simulink model "SW_Avionic"  (R2020a)
settings: Solver=FixedStepAuto  StartTime=0.0  StopTime=inf  FixedStep=0.01  RelTol=1e-3  EnableMultiTasking=on
libraries: bbblueCommlib x31, svdutilitieslib x13, bbblueBasicLib x6, bbblueSensorLib x3, simulink x1
settings Model: ExtModeTrigDuration=100  Creator=sokserey  LastModifiedBy=ASUS
settings SolverCC: PositivePriorityOrder=on  AutoInsertRateTranBlk=on
settings OptimizationCC: EnhancedBackFolding=on  PassReuseOutputArgsAs=Individual arguments  ZeroExternalMemoryAtStartup=off  ZeroInternalMemoryAtStartup=off  MaxStackSize=64  OptimizeBlockOrder=speed  DifferentSizesBufferReuse=on  OptimizationCustomize=off  EfficientTunableParamExpr=on
settings DebuggingCC: ParameterTunabilityLossMsg=error  SFMachineParentedDataDiag=error
settings HardwareCC: ProdBitPerPointer=32  ProdBitPerSizeT=32  ProdBitPerPtrDiffT=32  ProdLargestAtomicInteger=Long  ProdLargestAtomicFloat=Double  ProdWordSize=32  ProdHWDeviceType=ARM Compatible->ARM Cortex
settings SFSimCC: MATLABDynamicMemAlloc=off
settings RTWCC: SystemTargetFile=ert.tlc  HardwareBoard=BeagleBone Blue  TemplateMakefile=ert_default_tmf  Toolchain=GNU GCC BeagleBone Blue
settings CodeAppCC: ForceParamTrailComments=on  IgnoreCustomStorageClasses=off  OperatorAnnotations=on  SimulinkDataObjDesc=on  SFDataObjDesc=on  InsertBlockDesc=on
settings ERTTargetCC: SupportContinuousTime=on  SupportVariableSizeSignals=on

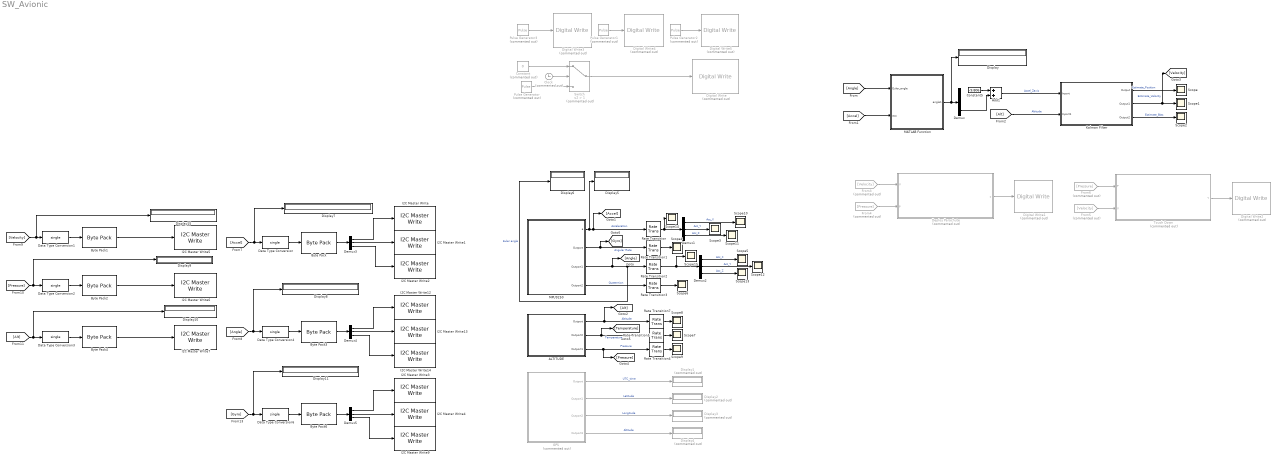
== system SW_Avionic ==
  "ALTITUDE " : Subsystem
  Add1 : Sum
  Byte Pack{,1..4,6} (6 alike) : svdutilitieslib/Byte Pack  maskPackedDataType=uint8  datatypes={'single'}  byteAlign=1  blockPlatform=arduinoert
      settings: SourceProductBaseCode=ARDUINO,ML_ARDUINO,ECCORTEXA,ECCORTEXR,SC_BEAGLEBONE_BLUE,EC_FREEDOM_BOARD,EC_FRDM_K64F,INTEL_BLOCKSET,MICROBIT,NUCLEO,PX4AUTOPILOTS,RASPPIIO,STMICRODIS,TIC2000,XILINX_BLOCKSET
  Clock : Clock  Commented=on
  Constant : Constant  Commented=on  Value=0
  Constant5 : Constant  Value=-9.806
  Data Type Conversion{,1..4,6} (6 alike) : DataTypeConversion  OutDataTypeStr=single
  Demux{,1..5} (6 alike) : Demux  Outputs=3
  "Deploy Parachute " : Stateflow chart  Commented=on  TreatAsAtomicUnit=on
  Digital Write : bbblueBasicLib/Digital Write  Commented=on  GPIOSelect=GPIO3_17  Pin=49  Direction=output
      settings: SourceProductBaseCode=SC_BEAGLEBONE_BLUE
  Digital Write1 : bbblueBasicLib/Digital Write  Commented=on  GPIOSelect=GPIO3_2  Pin=49  Direction=output
      settings: SourceProductBaseCode=SC_BEAGLEBONE_BLUE
  Digital Write2 : bbblueBasicLib/Digital Write  Commented=on  GPIOSelect=GPIO3_1  Pin=49  Direction=output
      settings: SourceProductBaseCode=SC_BEAGLEBONE_BLUE
  Digital Write3 : bbblueBasicLib/Digital Write  Commented=on  GPIOSelect=GPIO1_25  Pin=49  Direction=output
      settings: SourceProductBaseCode=SC_BEAGLEBONE_BLUE
  Digital Write4 : bbblueBasicLib/Digital Write  Commented=on  GPIOSelect=GPIO1_17  Pin=49  Direction=output
      settings: SourceProductBaseCode=SC_BEAGLEBONE_BLUE
  Digital Write5 : bbblueBasicLib/Digital Write  Commented=on  GPIOSelect=GPIO3_20  Pin=49  Direction=output
      settings: SourceProductBaseCode=SC_BEAGLEBONE_BLUE
  Display{,5..11,15} (9 alike) : Display
  Display{1..4} (4 alike) : Display  Commented=on
  From3 : From  Commented=on  GotoTag=Velocity
  From4 : From  Commented=on  GotoTag=Pressure
  From5 : From  Commented=on  GotoTag=Velocity
  From6 : From  Commented=on  GotoTag=Pressure
  GPS : Subsystem  Commented=on
  I2C Master Write{,1..7,9,12..14} (12 alike) : bbblueCommlib/I2C Master Write  I2CModule=1  Mode=Master  SlaveAddress=8  SlaveByteOrder=BigEndian  Direction=Transmitter  RegisterAddressMode=off  RegisterAddress=0  SlaveDataType=uint8  DataLength=1  NoAck=off  RepeatedStart=off  OutputStatus=off
      settings: SourceProductBaseCode=SC_BEAGLEBONE_BLUE
  "Kalman Filter " : Subsystem
  MATLAB Function : MATLAB Function  TreatAsAtomicUnit=on
  MPU9250 : Subsystem
  Pulse Generator : DiscretePulseGenerator  Commented=on  PulseType=Time based  Period=0.5  PulseWidth=50  VectorParams1D=off
  Pulse Generator1 : DiscretePulseGenerator  Commented=on  PulseType=Time based  Period=1  PulseWidth=33  PhaseDelay=0.33
  Pulse Generator2 : DiscretePulseGenerator  Commented=on  PulseType=Time based  Period=1  PulseWidth=33  PhaseDelay=0.66  VectorParams1D=off
  Pulse Generator3 : DiscretePulseGenerator  Commented=on  PulseType=Time based  Period=1  PulseWidth=33  VectorParams1D=off
  Rate Transition{,1..3} (4 alike) : RateTransition  OutPortSampleTime=0.01
  Rate Transition4 : RateTransition  OutPortSampleTime=0.1
  Rate Transition5 : RateTransition  OutPortSampleTime=0.1
  Rate Transition7 : RateTransition  OutPortSampleTime=0.1
  Scope{,1..15} (16 alike) : Scope
  Switch : Switch  Commented=on  Criteria=u2 > Threshold  Threshold=1
  "Touch Down " : Stateflow chart  Commented=on  TreatAsAtomicUnit=on
  wires:
  Clock/1 -> Switch/2
  Constant/1 -> Switch/1
  Pulse Generator/1 -> Switch/3
  Switch/1 -> Digital Write/1
  MPU9250/3(Outport1) -> Display6/1, Rate Transition2/1, [Angle]  "Euler angle"
  MPU9250/2(Outport) -> [Gyro], Rate Transition1/1  "Angular Rate"
  MPU9250/1(a) -> Rate Transition/1, [Accel], Display5/1  "Acceleration"
  MPU9250/4(Outport2) -> Rate Transition3/1  "Quaternion"
  "ALTITUDE "/3(Outport1) -> Rate Transition4/1, [Pressure]  "Pressure"
  Pulse Generator2/1 -> Digital Write5/1
  Pulse Generator1/1 -> Digital Write4/1
  Pulse Generator3/1 -> Digital Write3/1
  Constant5/1 -> Add1/1
  Add1/1 -> "Kalman Filter "/1(Inport)  "Accel_Zaxis"
  "Kalman Filter "/1(Output) -> Scope/1  "Estimate_Position"
  "Kalman Filter "/2(Output1) -> [Velocity], Scope1/1  "Estimate_Velocity"
  "Kalman Filter "/3(Output2) -> Scope2/1  "Estimate_Bias"
  [Angle] -> MATLAB Function/1(Euler_angle)
  [Accel] -> MATLAB Function/2(acc)
  MATLAB Function/1(angle1) -> Display/1, Demux/1
  Demux/3 -> Add1/2
  [Alt] -> "Kalman Filter "/2(Inport1)  "Altitude"
  GPS/1(Outport) -> Display1/1  "UTC_time"
  GPS/2(Outport1) -> Display2/1  "Latitude"
  GPS/3(Outport2) -> Display3/1  "Longitude"
  GPS/4(Outport3) -> Display4/1  "Altitude"
  Rate Transition1/1 -> Scope4/1
  Rate Transition3/1 -> Scope6/1
  Rate Transition7/1 -> Scope8/1
  Rate Transition5/1 -> Scope7/1
  Rate Transition4/1 -> Scope9/1
  "ALTITUDE "/1(Outport) -> [Alt], Rate Transition7/1  "Altitude"
  "ALTITUDE "/2(Outport2) -> [Temperature], Rate Transition5/1  "Temperature"
  "Deploy Parachute "/1(y) -> Digital Write1/1
  From3/1 -> "Deploy Parachute "/1(V)
  From4/1 -> "Deploy Parachute "/2(P)
  From5/1 -> "Touch Down "/2(V)
  From6/1 -> "Touch Down "/1(P)
  "Touch Down "/1(Y) -> Digital Write2/1
  Rate Transition/1 -> Scope14/1, Demux1/1
  Demux1/1 -> Scope10/1  "Acc_X"
  Demux1/2 -> Scope3/1  "Acc_Y"
  Demux1/3 -> Scope11/1  "Acc_Z"
  Rate Transition2/1 -> Scope15/1, Demux2/1
  Demux2/1 -> Scope5/1  "Acc_X"
  Demux2/3 -> Scope13/1  "Acc_Z"
  Demux2/2 -> Scope12/1  "Acc_Y"
  Demux3/3 -> I2C Master Write2/1
  Data Type Conversion4/1 -> Byte Pack3/1
  Byte Pack/1 -> Demux3/1
  Demux3/2 -> I2C Master Write1/1
  Demux4/3 -> I2C Master Write14/1
  Byte Pack3/1 -> Demux4/1
  Demux4/1 -> I2C Master Write12/1
  Demux4/2 -> I2C Master Write13/1
  Data Type Conversion/1 -> Byte Pack/1
  Demux3/1 -> I2C Master Write/1
  [Accel] -> Display7/1, Data Type Conversion/1
  [Angle] -> Display8/1, Data Type Conversion4/1
  Data Type Conversion1/1 -> Byte Pack1/1
  [Velocity] -> Display15/1, Data Type Conversion1/1
  Data Type Conversion2/1 -> Byte Pack2/1
  Byte Pack2/1 -> I2C Master Write6/1
  [Pressure] -> Display9/1, Data Type Conversion2/1
  Byte Pack4/1 -> I2C Master Write7/1
  [Alt] -> Display10/1, Data Type Conversion3/1
  Data Type Conversion3/1 -> Byte Pack4/1
  Byte Pack1/1 -> I2C Master Write5/1
  Demux5/1 -> I2C Master Write3/1
  [Gyro] -> Display11/1, Data Type Conversion6/1
  Byte Pack6/1 -> Demux5/1
  Demux5/2 -> I2C Master Write4/1
  Demux5/3 -> I2C Master Write9/1
  Data Type Conversion6/1 -> Byte Pack6/1

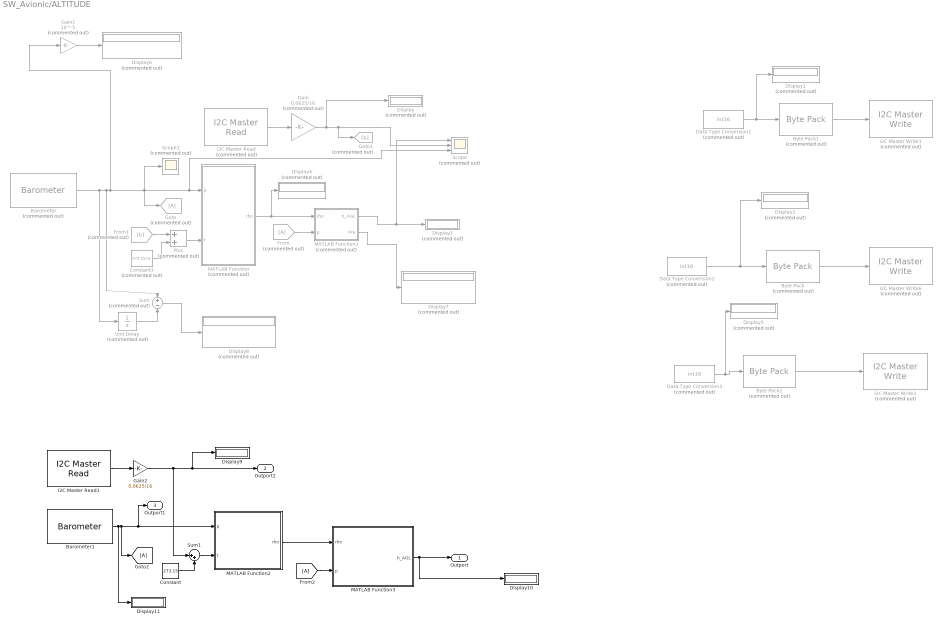
== system SW_Avionic/ALTITUDE  ==
  Barometer : bbblueSensorLib/Barometer  Commented=on  OSRSelection=16  IIRFilterCoeff=16  SampleTime=0.01
      settings: SourceProductBaseCode=SC_BEAGLEBONE_BLUE
  Barometer1 : bbblueSensorLib/Barometer  OSRSelection=16  IIRFilterCoeff=16  SampleTime=0.01
      settings: SourceProductBaseCode=SC_BEAGLEBONE_BLUE
  Byte Pack : svdutilitieslib/Byte Pack  Commented=on  maskPackedDataType=uint8  datatypes={'int16'}  byteAlign=1  blockPlatform=arduinoert
      settings: SourceProductBaseCode=ARDUINO,ML_ARDUINO,ECCORTEXA,ECCORTEXR,SC_BEAGLEBONE_BLUE,EC_FREEDOM_BOARD,EC_FRDM_K64F,INTEL_BLOCKSET,MICROBIT,NUCLEO,PX4AUTOPILOTS,RASPPIIO,STMICRODIS,TIC2000,XILINX_BLOCKSET
  Byte Pack1 : svdutilitieslib/Byte Pack  Commented=on  maskPackedDataType=uint8  datatypes={'int16'}  byteAlign=1  blockPlatform=arduinoert
      settings: SourceProductBaseCode=ARDUINO,ML_ARDUINO,ECCORTEXA,ECCORTEXR,SC_BEAGLEBONE_BLUE,EC_FREEDOM_BOARD,EC_FRDM_K64F,INTEL_BLOCKSET,MICROBIT,NUCLEO,PX4AUTOPILOTS,RASPPIIO,STMICRODIS,TIC2000,XILINX_BLOCKSET
  Byte Pack2 : svdutilitieslib/Byte Pack  Commented=on  maskPackedDataType=uint8  datatypes={'int16'}  byteAlign=1  blockPlatform=arduinoert
      settings: SourceProductBaseCode=ARDUINO,ML_ARDUINO,ECCORTEXA,ECCORTEXR,SC_BEAGLEBONE_BLUE,EC_FREEDOM_BOARD,EC_FRDM_K64F,INTEL_BLOCKSET,MICROBIT,NUCLEO,PX4AUTOPILOTS,RASPPIIO,STMICRODIS,TIC2000,XILINX_BLOCKSET
  Constant : Constant  Value=273.15
  Constant3 : Constant  Commented=on  Value=273.15+6
  Data Type Conversion1 : DataTypeConversion  Commented=on  OutDataTypeStr=int16
  Data Type Conversion2 : DataTypeConversion  Commented=on  OutDataTypeStr=int16
  Data Type Conversion3 : DataTypeConversion  Commented=on  OutDataTypeStr=int16
  Display{,1..8} (9 alike) : Display  Commented=on
  Display10 : Display
  Display11 : Display
  Display9 : Display
  From : From  Commented=on
  From1 : From  Commented=on  GotoTag=b
  Gain : Gain  Commented=on  Gain=0.0625/16  OutDataTypeStr=single
  Gain1 : Gain  Commented=on  Gain=10^-5
  Gain2 : Gain  Gain=0.0625/16  OutDataTypeStr=single
  Goto : Goto  Commented=on
  Goto1 : Goto  Commented=on  GotoTag=b
  I2C Master Read : bbblueCommlib/I2C Master Read  Commented=on  I2CModule=1  Mode=Master  SlaveAddress=hex2dec('48')  SlaveByteOrder=BigEndian  Direction=Receiver  RegisterAddressMode=off  RegisterAddress=0  SlaveDataType=int16  DataLength=1  NoAck=off  RepeatedStart=off  OutputStatus=off  SampleTime=0.1
      settings: SourceProductBaseCode=SC_BEAGLEBONE_BLUE
  I2C Master Read1 : bbblueCommlib/I2C Master Read  I2CModule=1  Mode=Master  SlaveAddress=hex2dec('48')  SlaveByteOrder=BigEndian  Direction=Receiver  RegisterAddressMode=off  RegisterAddress=0  SlaveDataType=int16  DataLength=1  NoAck=off  RepeatedStart=off  OutputStatus=off  SampleTime=0.1
      settings: SourceProductBaseCode=SC_BEAGLEBONE_BLUE
  I2C Master Write1 : bbblueCommlib/I2C Master Write  Commented=on  I2CModule=1  Mode=Master  SlaveAddress=8  SlaveByteOrder=BigEndian  Direction=Transmitter  RegisterAddressMode=off  RegisterAddress=0  SlaveDataType=uint8  DataLength=1  NoAck=off  RepeatedStart=off  OutputStatus=off
      settings: SourceProductBaseCode=SC_BEAGLEBONE_BLUE
  I2C Master Write2 : bbblueCommlib/I2C Master Write  Commented=on  I2CModule=1  Mode=Master  SlaveAddress=8  SlaveByteOrder=BigEndian  Direction=Transmitter  RegisterAddressMode=off  RegisterAddress=0  SlaveDataType=uint8  DataLength=1  NoAck=off  RepeatedStart=off  OutputStatus=off
      settings: SourceProductBaseCode=SC_BEAGLEBONE_BLUE
  I2C Master Write6 : bbblueCommlib/I2C Master Write  Commented=on  I2CModule=1  Mode=Master  SlaveAddress=8  SlaveByteOrder=BigEndian  Direction=Transmitter  RegisterAddressMode=off  RegisterAddress=0  SlaveDataType=uint8  DataLength=1  NoAck=off  RepeatedStart=off  OutputStatus=off
      settings: SourceProductBaseCode=SC_BEAGLEBONE_BLUE
  MATLAB Function : MATLAB Function  Commented=on  TreatAsAtomicUnit=on
  MATLAB Function1 : MATLAB Function  Commented=on  TreatAsAtomicUnit=on
  MATLAB Function2 : MATLAB Function  TreatAsAtomicUnit=on
  MATLAB Function3 : MATLAB Function  TreatAsAtomicUnit=on
  Plus : Sum  Commented=on
  Scope : Scope  Commented=on  NumInputPorts=3
  Scope1 : Scope  Commented=on
  Sum : Sum  Commented=on  Inputs=+-
  Sum1 : Sum  Inputs=|++
  Unit Delay : UnitDelay  Commented=on  SampleTime=-1  HasFrameUpgradeWarning=on
  Outport : Outport
  Outport2 : Outport  Port=2
  Outport1 : Outport  Port=3
  wires:
  I2C Master Read/1 -> Gain/1
  Plus/1 -> MATLAB Function/2(t)
  Gain/1 -> Display/1, Scope/2, Goto1/1
  MATLAB Function/1(rho) -> Display4/1, MATLAB Function1/1(rho)
  Constant3/1 -> Plus/2
  From/1 -> MATLAB Function1/2(p)
  From1/1 -> Plus/1
  MATLAB Function1/1(h_AGL) -> Display3/1, Scope/1
  Data Type Conversion2/1 -> Byte Pack/1, Display2/1
  Data Type Conversion1/1 -> Display1/1, Byte Pack1/1
  Byte Pack/1 -> I2C Master Write6/1
  Byte Pack1/1 -> I2C Master Write1/1
  Data Type Conversion3/1 -> Display5/1, Byte Pack2/1
  Byte Pack2/1 -> I2C Master Write2/1
  Barometer/1 -> Scope/3, MATLAB Function/1(p), Scope1/1, Goto/1, Gain1/1, Sum/1, Unit Delay/1
  Gain1/1 -> Display6/1
  MATLAB Function1/2(Pre) -> Display7/1
  Unit Delay/1 -> Sum/2
  Sum/1 -> Display8/1
  I2C Master Read1/1 -> Gain2/1
  Barometer1/1 -> Display11/1, MATLAB Function2/1(p), Outport1/1, [A]
  Gain2/1 -> Sum1/1, Display9/1, Outport2/1
  MATLAB Function2/1(rho) -> MATLAB Function3/1(rho)
  [A] -> MATLAB Function3/2(p)
  MATLAB Function3/1(h_AGL) -> Display10/1, Outport/1
  Sum1/1 -> MATLAB Function2/2(t)
  Constant/1 -> Sum1/2

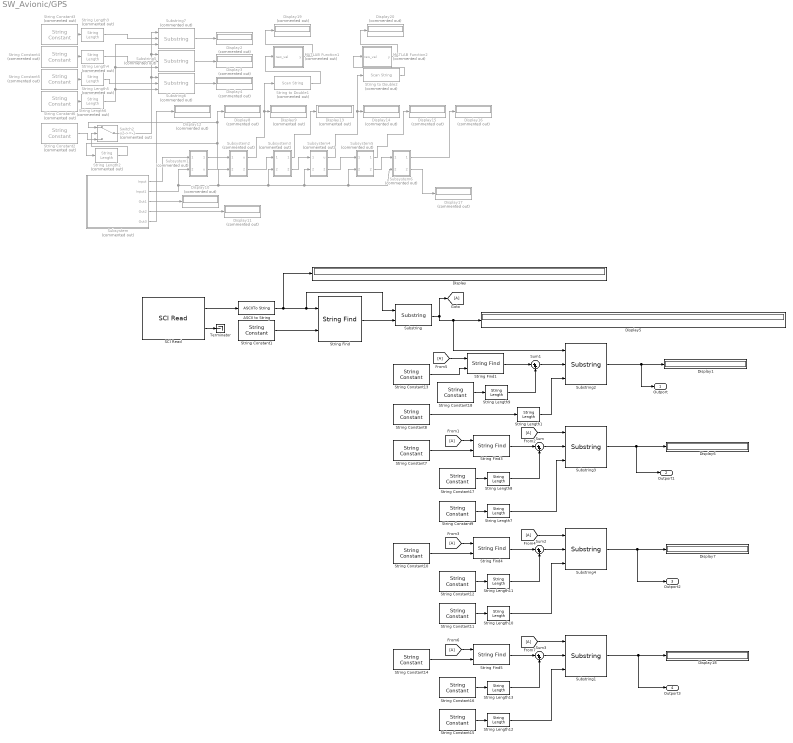
== system SW_Avionic/GPS ==
  ASCII to String : ASCIIToString
  Display{,1,5..7,18} (6 alike) : Display
  Display{2..4,8..17,19..20} (15 alike) : Display  Commented=on
  MATLAB Function1 : MATLAB Function  Commented=on  TreatAsAtomicUnit=on
  MATLAB Function2 : MATLAB Function  Commented=on  TreatAsAtomicUnit=on
  SCI Read : bbblueCommlib/SCI Read  SCIModule=/dev/ttyO2  BaudrateOptions=9600  Parity=None  StopbitOptions=1  Baudrate=uint32(9600)  StopBits=1  HardwareFlowControl=None  ByteOrder=LittleEndian  DataType=uint8  DataLength=150  OutputStatus=on  SampleTime=0.1
      settings: SourceProductBaseCode=SC_BEAGLEBONE_BLUE
  String Constant1 : StringConstant  String="\"$GPGGA\""
  String Constant{7,10,13..14} (4 alike) : StringConstant  String="\",\""
  String Constant11 : StringConstant  String="\"hhhhhhhhhh\""
  String Constant12 : StringConstant  String="\"123456789101111111111111\""
  String Constant15 : StringConstant  String="\"hhhh\""
  String Constant16 : StringConstant  String="\"123456789101111111111111111111111111111111111111\""
  String Constant17 : StringConstant  String="\"12345678910\""
  String Constant18 : StringConstant  String="\"1\""
  String Constant2 : StringConstant  Commented=on  String="\"000000\""
  String Constant3 : StringConstant  Commented=on  String="\"0\""
  String Constant4 : StringConstant  Commented=on  String="\"000\""
  String Constant5 : StringConstant  Commented=on  String="\"00000\""
  String Constant6 : StringConstant  Commented=on  String="\"00\""
  String Constant8 : StringConstant  String="\"hhhhhh\""
  String Constant9 : StringConstant  String="\"hhhhhhhhhh\""
  String Find{,1,3..5} (5 alike) : StringFind
  String Length{1,7,10,12} (4 alike) : StringLength
  String Length{8..9,11,13} (4 alike) : StringLength  OutDataTypeStr=int32
  String Length{2..6} (5 alike) : StringLength  Commented=on
  String to Double1 : ScanString  Commented=on  Format="\"%lf\""
  String to Double2 : ScanString  Commented=on  Format="\"%lf\""
  Substring : Substring  StringFromIdxToEnd=on
  Substring{1..4} (4 alike) : Substring
  Substring5 : Substring  Commented=on
  Substring6 : Substring  Commented=on
  Substring7 : Substring  Commented=on
  Subsystem : Subsystem  Commented=on
  Subsystem1 : Subsystem  Commented=on
  Subsystem2 : Subsystem  Commented=on
  Subsystem3 : Subsystem  Commented=on
  Subsystem4 : Subsystem  Commented=on
  Subsystem5 : Subsystem  Commented=on
  Subsystem6 : Subsystem  Commented=on
  Sum{,1..3} (4 alike) : Sum  Inputs=|++
  Switch2 : Switch  Commented=on  Threshold=1
  Terminator : Terminator
  Outport : Outport
  Outport1 : Outport  Port=2
  Outport2 : Outport  Port=3
  Outport3 : Outport  Port=4
  wires:
  Switch2/1 -> Substring6/1, Substring5/1, Substring7/1
  String Length6/1 -> Substring6/3, Substring7/3, Substring5/3
  String Length4/1 -> Substring5/2
  String Length3/1 -> Substring7/2
  Subsystem5/1(Out1) -> Display15/1
  Subsystem/5(Out3) -> Display12/1
  Substring6/1 -> Display4/1
  String Constant5/1 -> String Length5/1
  String Constant4/1 -> String Length4/1
  String Length2/1 -> Switch2/2
  String Constant2/1 -> Switch2/3
  String Constant3/1 -> String Length3/1
  MATLAB Function2/1(y) -> Display20/1
  String to Double2/1 -> MATLAB Function2/1(raw_val)
  Subsystem6/2(Out2) -> Display17/1
  Subsystem3/1(Out1) -> Display13/1
  Subsystem3/2(Out2) -> Subsystem4/1(In1)
  Subsystem2/1(u) -> String to Double1/1, Display9/1
  Subsystem4/1(u) -> String to Double2/1, Display14/1
  Subsystem5/2(Out2) -> Subsystem6/1(In1)
  Subsystem4/2(Out2) -> Subsystem5/1(In1)
  String Length5/1 -> Substring6/2
  Subsystem/4(Out2) -> Display11/1
  String Constant6/1 -> String Length6/1
  MATLAB Function1/1(y) -> Display19/1
  Subsystem1/1(Out1) -> Subsystem2/1(In1)
  String to Double1/1 -> MATLAB Function1/1(raw_val)
  Subsystem/1(Input) -> Subsystem1/1(Input)
  Subsystem6/1(Out1) -> Display16/1
  Subsystem/3(Out1) -> Display10/1
  Subsystem/2(Input1) -> Subsystem1/2(Input1), Subsystem6/2(Input1), Subsystem5/2(Input1), Subsystem4/2(Input1), Subsystem3/2(Input1), Subsystem2/2(Input1)
  Subsystem2/2(Out2) -> Subsystem3/1(In1)
  Subsystem1/2(u) -> String Length2/1, Switch2/1, Display8/1
  Substring5/1 -> Display3/1
  Substring7/1 -> Display2/1
  [A] -> String Find3/1
  String Constant9/1 -> String Length7/1
  String Length7/1 -> Substring3/3
  Substring3/1 -> Outport1/1, Display6/1
  Substring1/1 -> Outport3/1, Display18/1
  String Constant16/1 -> String Length13/1
  [A] -> Substring1/1
  String Constant18/1 -> String Length9/1
  String Find5/1 -> Sum3/1
  [A] -> String Find5/1
  [A] -> Substring3/1
  String Find4/1 -> Sum2/1
  String Length10/1 -> Substring4/3
  String Find3/1 -> Sum/1
  String Length12/1 -> Substring1/3
  String Constant10/1 -> String Find4/2
  String Length11/1 -> Sum2/2
  [A] -> String Find4/1
  String Constant11/1 -> String Length10/1
  [A] -> Substring4/1
  String Constant12/1 -> String Length11/1
  String Constant13/1 -> String Find1/2
  [A] -> String Find1/1
  Sum2/1 -> Substring4/2
  String Length9/1 -> Sum1/2
  String Find1/1 -> Sum1/1
  String Length8/1 -> Sum/2
  String Length1/1 -> Substring2/3
  String Constant1/1 -> String Find/2
  Substring2/1 -> Outport/1, Display1/1
  String Constant15/1 -> String Length12/1
  Sum1/1 -> Substring2/2
  String Constant8/1 -> String Length1/1
  SCI Read/1 -> ASCII to String/1
  String Constant7/1 -> String Find3/2
  ASCII to String/1 -> Substring/1, String Find/1, Display/1
  Substring4/1 -> Outport2/1, Display7/1
  String Find/1 -> Substring/2
  Sum3/1 -> Substring1/2
  Substring/1 -> Substring2/1, Display5/1, [A]
  Sum/1 -> Substring3/2
  String Length13/1 -> Sum3/2
  String Constant14/1 -> String Find5/2
  String Constant17/1 -> String Length8/1
  SCI Read/2 -> Terminator/1

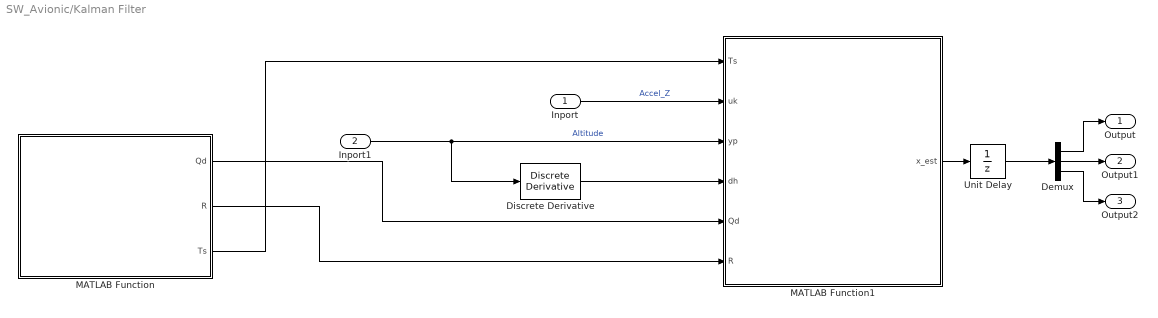
== system SW_Avionic/Kalman Filter  ==
  Inport : Inport
  Inport1 : Inport  Port=2
  Demux : Demux  Outputs=3
  Discrete Derivative : simulink/Discrete/Discrete Derivative  gainval=1.0  ICPrevScaledInput=0.0  OutMin=[]  OutMax=[]  OutDataType=fixdt(1, 16)  OutScaling=2^-10  DoSatur=off
  MATLAB Function : MATLAB Function  TreatAsAtomicUnit=on
  MATLAB Function1 : MATLAB Function  TreatAsAtomicUnit=on
  Unit Delay : UnitDelay  InitialCondition=[0;0;0]  SampleTime=-1  HasFrameUpgradeWarning=on
  Output : Outport
  Output1 : Outport  Port=2
  Output2 : Outport  Port=3
  wires:
  MATLAB Function/2(R) -> MATLAB Function1/6(R)
  MATLAB Function1/1(x_est) -> Unit Delay/1
  MATLAB Function/3(Ts) -> MATLAB Function1/1(Ts)
  Inport/1 -> MATLAB Function1/2(uk)  "Accel_Z"
  MATLAB Function/1(Qd) -> MATLAB Function1/5(Qd)
  Inport1/1 -> Discrete Derivative/1, MATLAB Function1/3(yp)  "Altitude"
  Unit Delay/1 -> Demux/1
  Demux/1 -> Output/1
  Demux/2 -> Output1/1
  Discrete Derivative/1 -> MATLAB Function1/4(dh)
  Demux/3 -> Output2/1

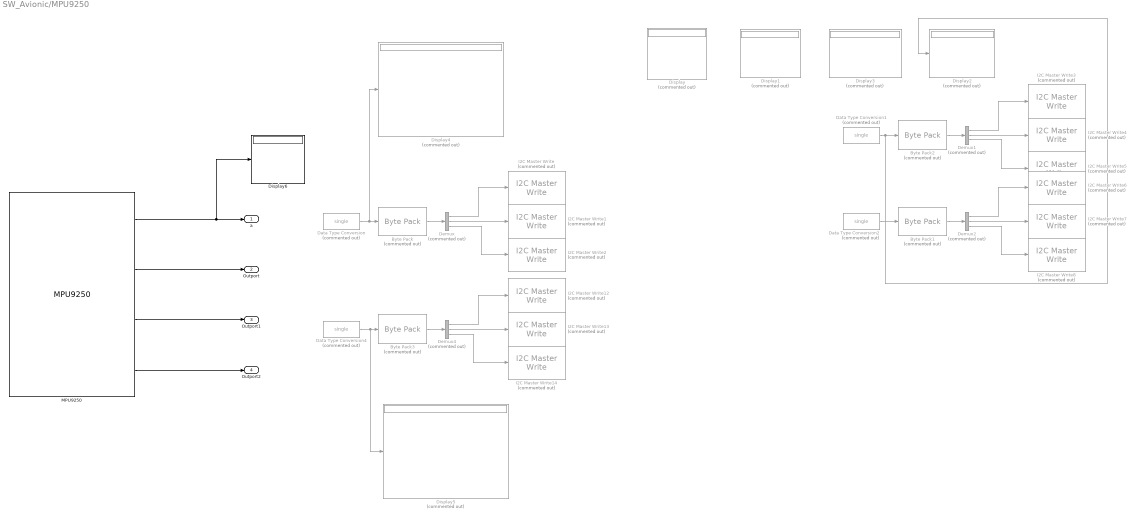
== system SW_Avionic/MPU9250 ==
  Byte Pack{,1..3} (4 alike) : svdutilitieslib/Byte Pack  Commented=on  maskPackedDataType=uint8  datatypes={'single'}  byteAlign=1  blockPlatform=arduinoert
      settings: SourceProductBaseCode=ARDUINO,ML_ARDUINO,ECCORTEXA,ECCORTEXR,SC_BEAGLEBONE_BLUE,EC_FREEDOM_BOARD,EC_FRDM_K64F,INTEL_BLOCKSET,MICROBIT,NUCLEO,PX4AUTOPILOTS,RASPPIIO,STMICRODIS,TIC2000,XILINX_BLOCKSET
  Data Type Conversion{,1..2,4} (4 alike) : DataTypeConversion  Commented=on  OutDataTypeStr=single
  Demux{,1..2,4} (4 alike) : Demux  Commented=on  Outputs=3
  Display{,1..5} (6 alike) : Display  Commented=on
  Display6 : Display
  I2C Master Write{,1..8,12..14} (12 alike) : bbblueCommlib/I2C Master Write  Commented=on  I2CModule=1  Mode=Master  SlaveAddress=8  SlaveByteOrder=BigEndian  Direction=Transmitter  RegisterAddressMode=off  RegisterAddress=0  SlaveDataType=uint8  DataLength=1  NoAck=off  RepeatedStart=off  OutputStatus=off
      settings: SourceProductBaseCode=SC_BEAGLEBONE_BLUE
  MPU9250 : bbblueSensorLib/MPU9250  OperationMode=DMP  Accel=on  AngularRate=on  Ak8963Field=off  EulerAngles=on  Quat=on  AccelRange=16G  Acceldlpf=1  GyroRange=250 dps  Gyrodlpf=1  DmpOdr=200 Hz  SampleTime=0.01
      settings: SourceProductBaseCode=SC_BEAGLEBONE_BLUE
  a : Outport
  Outport : Outport  Port=2
  Outport1 : Outport  Port=3
  Outport2 : Outport  Port=4
  wires:
  Demux/1 -> I2C Master Write/1
  Demux/2 -> I2C Master Write1/1
  Byte Pack/1 -> Demux/1
  Demux/3 -> I2C Master Write2/1
  MPU9250/2 -> Outport/1
  MPU9250/3 -> Outport1/1
  MPU9250/4 -> Outport2/1
  Data Type Conversion/1 -> Display4/1, Byte Pack/1
  Demux4/1 -> I2C Master Write12/1
  Byte Pack3/1 -> Demux4/1
  Data Type Conversion4/1 -> Display5/1, Byte Pack3/1
  Demux4/2 -> I2C Master Write13/1
  Demux4/3 -> I2C Master Write14/1
  Demux1/3 -> I2C Master Write5/1
  Data Type Conversion1/1 -> Byte Pack2/1, Display2/1
  Byte Pack2/1 -> Demux1/1
  Demux1/1 -> I2C Master Write3/1
  Demux1/2 -> I2C Master Write4/1
  Demux2/3 -> I2C Master Write8/1
  Data Type Conversion2/1 -> Byte Pack1/1
  Byte Pack1/1 -> Demux2/1
  Demux2/1 -> I2C Master Write6/1
  Demux2/2 -> I2C Master Write7/1
  MPU9250/1 -> Display6/1, a/1

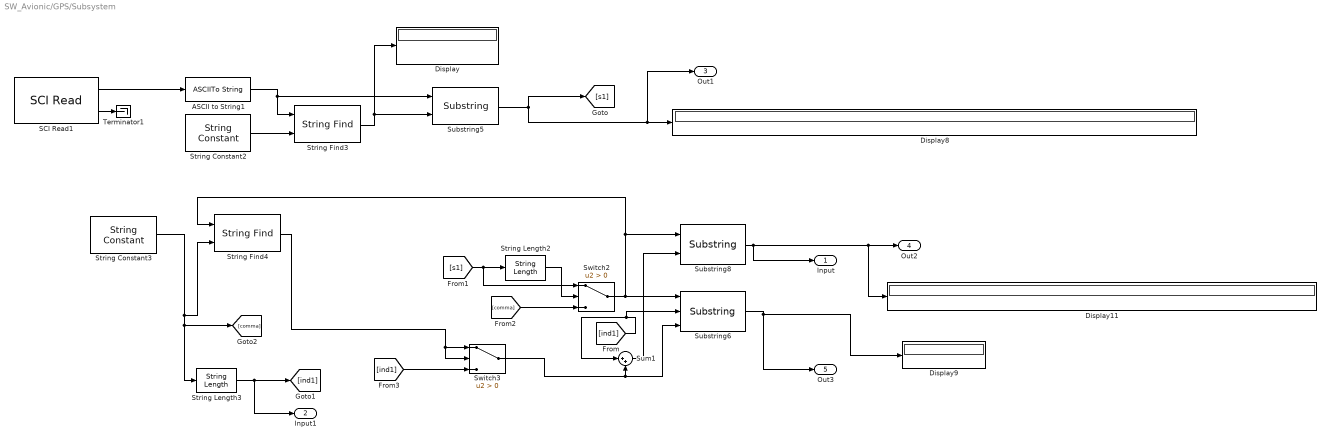
== system SW_Avionic/GPS/Subsystem ==
  ASCII to String1 : ASCIIToString
  Display{,8..9,11} (4 alike) : Display
  SCI Read1 : bbblueCommlib/SCI Read  SCIModule=/dev/ttyO1  BaudrateOptions=9600  Parity=None  StopbitOptions=1  Baudrate=uint32(9600)  StopBits=1  HardwareFlowControl=None  ByteOrder=LittleEndian  DataType=uint8  DataLength=100  OutputStatus=on  SampleTime=0.1
      settings: SourceProductBaseCode=SC_BEAGLEBONE_BLUE
  String Constant2 : StringConstant  String="\"$GPGGA\""
  String Constant3 : StringConstant  String="\",\""
  String Find3 : StringFind
  String Find4 : StringFind
  String Length2 : StringLength
  String Length3 : StringLength
  Substring5 : Substring  InheritMaximumLength=off  StringFromIdxToEnd=on
  Substring6 : Substring
  Substring8 : Substring  StringFromIdxToEnd=on
  Sum1 : Sum  Inputs=|++
  Switch2 : Switch  Criteria=u2 > Threshold
  Switch3 : Switch  Criteria=u2 > Threshold
  Terminator1 : Terminator
  Input : Outport
  Input1 : Outport  Port=2
  Out1 : Outport  Port=3
  Out2 : Outport  Port=4
  Out3 : Outport  Port=5
  wires:
  Sum1/1 -> Substring8/2
  Substring6/1 -> Out3/1, Display9/1
  [s1] -> Switch2/1, String Length2/1
  Switch3/1 -> Substring6/3, Sum1/2
  String Constant2/1 -> String Find3/2
  [comma] -> Switch2/3
  ASCII to String1/1 -> Substring5/1, String Find3/1
  String Find4/1 -> Switch3/2, Switch3/1
  Switch2/1 -> Substring8/1, String Find4/1, Substring6/1
  String Constant3/1 -> String Find4/2, String Length3/1, [comma]
  SCI Read1/2 -> Terminator1/1
  String Find3/1 -> Substring5/2, Display/1
  SCI Read1/1 -> ASCII to String1/1
  String Length2/1 -> Switch2/2
  Substring8/1 -> Input/1, Display11/1, Out2/1
  [ind1] -> Switch3/3
  [ind1] -> Sum1/1, Substring6/2
  Substring5/1 -> Out1/1, Display8/1, [s1]
  String Length3/1 -> Input1/1, [ind1]

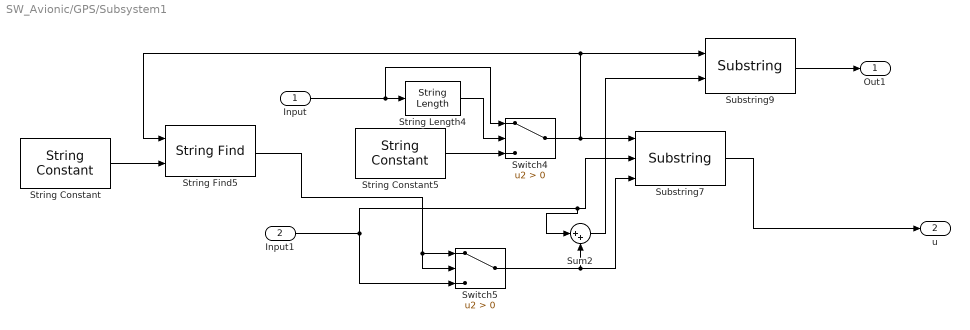
== system SW_Avionic/GPS/Subsystem1 ==
  Input : Inport
  Input1 : Inport  Port=2
  String Constant : StringConstant  String="\",\""
  String Constant5 : StringConstant  String="\"1\""
  String Find5 : StringFind
  String Length4 : StringLength
  Substring7 : Substring
  Substring9 : Substring  StringFromIdxToEnd=on
  Sum2 : Sum  Inputs=|++
  Switch4 : Switch  Criteria=u2 > Threshold
  Switch5 : Switch  Criteria=u2 > Threshold
  Out1 : Outport
  u : Outport  Port=2
  wires:
  Sum2/1 -> Substring9/2
  String Constant5/1 -> Switch4/3
  Substring9/1 -> Out1/1
  String Find5/1 -> Switch5/2, Switch5/1
  Switch4/1 -> Substring9/1, String Find5/1, Substring7/1
  String Length4/1 -> Switch4/2
  Input/1 -> Switch4/1, String Length4/1
  String Constant/1 -> String Find5/2
  Switch5/1 -> Sum2/2, Substring7/3
  Input1/1 -> Switch5/3, Substring7/2, Sum2/1
  Substring7/1 -> u/1

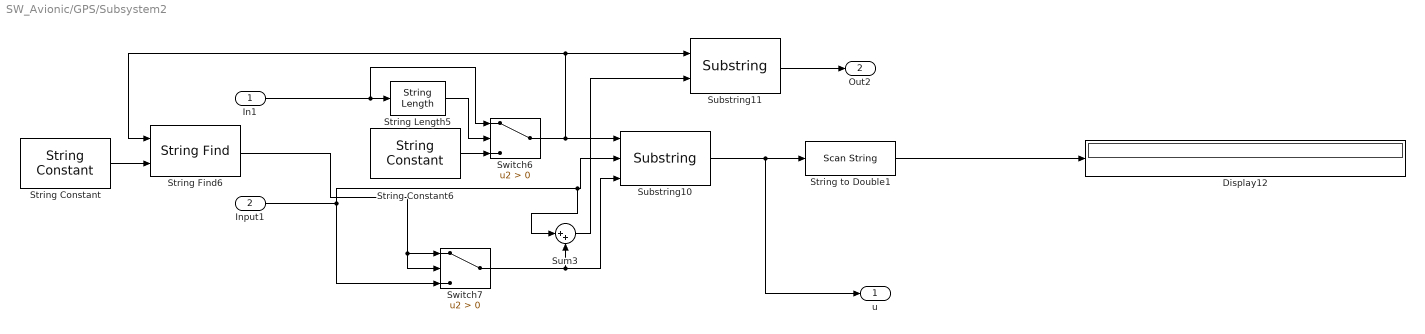
== system SW_Avionic/GPS/Subsystem2 ==
  In1 : Inport
  Input1 : Inport  Port=2
  Display12 : Display
  String Constant : StringConstant  String="\",\""
  String Constant6 : StringConstant  String="\"1\""
  String Find6 : StringFind
  String Length5 : StringLength
  String to Double1 : ScanString  Format="\"%lf\""
  Substring10 : Substring
  Substring11 : Substring  StringFromIdxToEnd=on
  Sum3 : Sum  Inputs=|++
  Switch6 : Switch  Criteria=u2 > Threshold
  Switch7 : Switch  Criteria=u2 > Threshold
  u : Outport
  Out2 : Outport  Port=2
  wires:
  String Constant/1 -> String Find6/2
  String to Double1/1 -> Display12/1
  String Find6/1 -> Switch7/1, Switch7/2
  Switch6/1 -> Substring10/1, String Find6/1, Substring11/1
  Switch7/1 -> Substring10/3, Sum3/2
  String Length5/1 -> Switch6/2
  Substring10/1 -> u/1, String to Double1/1
  String Constant6/1 -> Switch6/3
  In1/1 -> String Length5/1, Switch6/1
  Input1/1 -> Switch7/3, Substring10/2, Sum3/1
  Substring11/1 -> Out2/1
  Sum3/1 -> Substring11/2

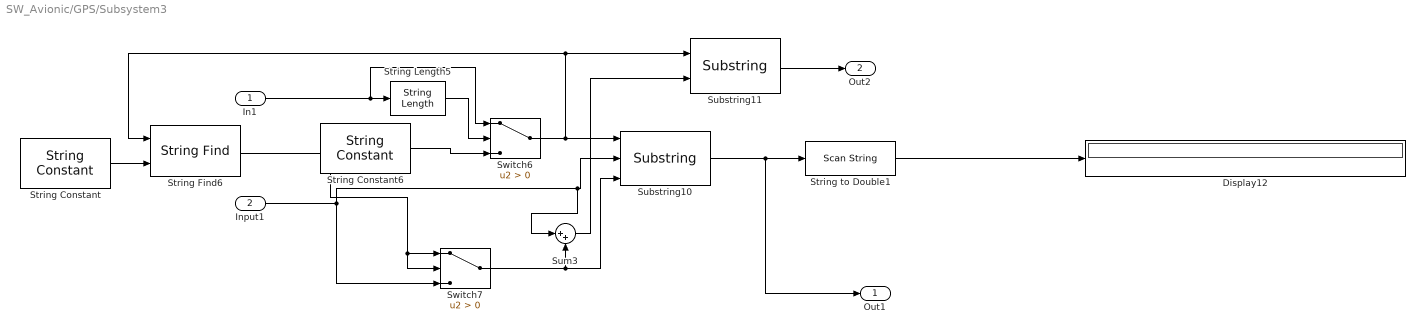
== system SW_Avionic/GPS/Subsystem3 ==
  In1 : Inport
  Input1 : Inport  Port=2
  Display12 : Display
  String Constant : StringConstant  String="\",\""
  String Constant6 : StringConstant  String="\"1\""
  String Find6 : StringFind
  String Length5 : StringLength
  String to Double1 : ScanString  Format="\"%lf\""
  Substring10 : Substring
  Substring11 : Substring  StringFromIdxToEnd=on
  Sum3 : Sum  Inputs=|++
  Switch6 : Switch  Criteria=u2 > Threshold
  Switch7 : Switch  Criteria=u2 > Threshold
  Out1 : Outport
  Out2 : Outport  Port=2
  wires:
  Sum3/1 -> Substring11/2
  Substring11/1 -> Out2/1
  Input1/1 -> Sum3/1, Substring10/2, Switch7/3
  In1/1 -> Switch6/1, String Length5/1
  String Constant6/1 -> Switch6/3
  Substring10/1 -> String to Double1/1, Out1/1
  String Length5/1 -> Switch6/2
  Switch7/1 -> Sum3/2, Substring10/3
  Switch6/1 -> Substring11/1, String Find6/1, Substring10/1
  String Find6/1 -> Switch7/2, Switch7/1
  String to Double1/1 -> Display12/1
  String Constant/1 -> String Find6/2

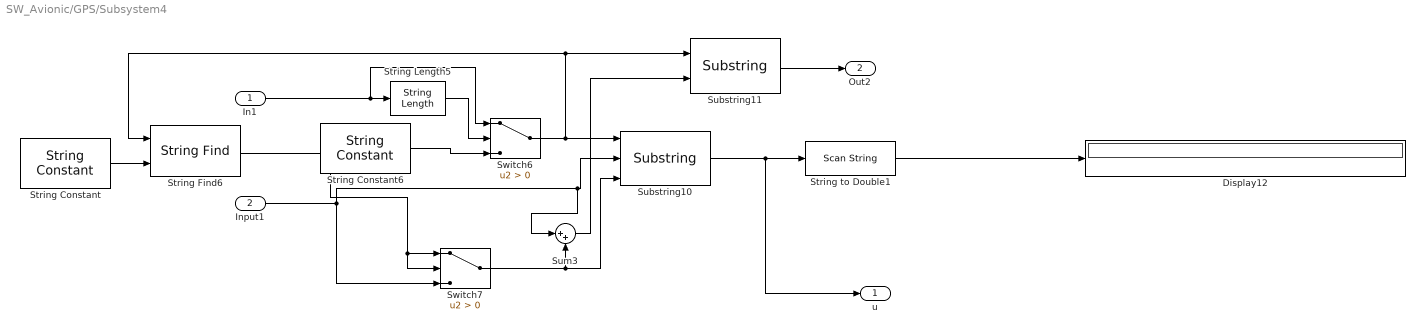
== system SW_Avionic/GPS/Subsystem4 ==
  In1 : Inport
  Input1 : Inport  Port=2
  Display12 : Display
  String Constant : StringConstant  String="\",\""
  String Constant6 : StringConstant  String="\"1\""
  String Find6 : StringFind
  String Length5 : StringLength
  String to Double1 : ScanString  Format="\"%lf\""
  Substring10 : Substring
  Substring11 : Substring  StringFromIdxToEnd=on
  Sum3 : Sum  Inputs=|++
  Switch6 : Switch  Criteria=u2 > Threshold
  Switch7 : Switch  Criteria=u2 > Threshold
  u : Outport
  Out2 : Outport  Port=2
  wires:
  String Constant/1 -> String Find6/2
  String to Double1/1 -> Display12/1
  String Find6/1 -> Switch7/1, Switch7/2
  Switch6/1 -> Substring10/1, String Find6/1, Substring11/1
  Switch7/1 -> Substring10/3, Sum3/2
  String Length5/1 -> Switch6/2
  Substring10/1 -> u/1, String to Double1/1
  String Constant6/1 -> Switch6/3
  In1/1 -> String Length5/1, Switch6/1
  Input1/1 -> Switch7/3, Substring10/2, Sum3/1
  Substring11/1 -> Out2/1
  Sum3/1 -> Substring11/2

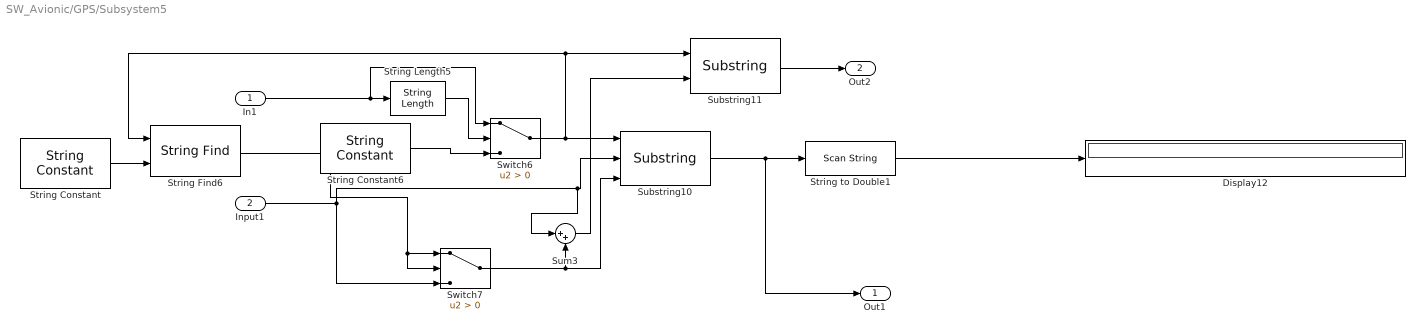
== system SW_Avionic/GPS/Subsystem5 ==
  In1 : Inport
  Input1 : Inport  Port=2
  Display12 : Display
  String Constant : StringConstant  String="\",\""
  String Constant6 : StringConstant  String="\"1\""
  String Find6 : StringFind
  String Length5 : StringLength
  String to Double1 : ScanString  Format="\"%lf\""
  Substring10 : Substring
  Substring11 : Substring  StringFromIdxToEnd=on
  Sum3 : Sum  Inputs=|++
  Switch6 : Switch  Criteria=u2 > Threshold
  Switch7 : Switch  Criteria=u2 > Threshold
  Out1 : Outport
  Out2 : Outport  Port=2
  wires:
  String Constant/1 -> String Find6/2
  String to Double1/1 -> Display12/1
  String Find6/1 -> Switch7/1, Switch7/2
  Switch6/1 -> Substring10/1, String Find6/1, Substring11/1
  Switch7/1 -> Substring10/3, Sum3/2
  String Length5/1 -> Switch6/2
  Substring10/1 -> Out1/1, String to Double1/1
  String Constant6/1 -> Switch6/3
  In1/1 -> String Length5/1, Switch6/1
  Input1/1 -> Switch7/3, Substring10/2, Sum3/1
  Substring11/1 -> Out2/1
  Sum3/1 -> Substring11/2

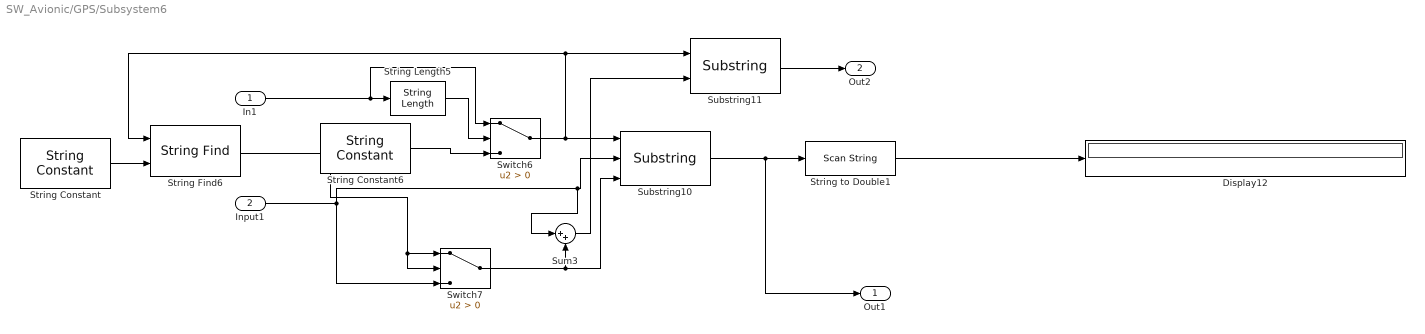
== system SW_Avionic/GPS/Subsystem6 ==
  In1 : Inport
  Input1 : Inport  Port=2
  Display12 : Display
  String Constant : StringConstant  String="\",\""
  String Constant6 : StringConstant  String="\"1\""
  String Find6 : StringFind
  String Length5 : StringLength
  String to Double1 : ScanString  Format="\"%lf\""
  Substring10 : Substring
  Substring11 : Substring  StringFromIdxToEnd=on
  Sum3 : Sum  Inputs=|++
  Switch6 : Switch  Criteria=u2 > Threshold
  Switch7 : Switch  Criteria=u2 > Threshold
  Out1 : Outport
  Out2 : Outport  Port=2
  wires:
  Sum3/1 -> Substring11/2
  Substring11/1 -> Out2/1
  Input1/1 -> Sum3/1, Substring10/2, Switch7/3
  In1/1 -> Switch6/1, String Length5/1
  String Constant6/1 -> Switch6/3
  Substring10/1 -> String to Double1/1, Out1/1
  String Length5/1 -> Switch6/2
  Switch7/1 -> Sum3/2, Substring10/3
  Switch6/1 -> Substring11/1, String Find6/1, Substring10/1
  String Find6/1 -> Switch7/2, Switch7/1
  String to Double1/1 -> Display12/1
  String Constant/1 -> String Find6/2

== matlab function SW_Avionic/MATLAB Function ==
  data: Euler_angle input; angle1 output; acc input
function angle1   = fcn(Euler_angle,acc)

% r = roll;
% p = pitch;
% y = yaw;
r = Euler_angle(1);
p = Euler_angle(2);
y = Euler_angle(3);

Rx = [1 0 0;
    0 cosd(r) sind(r);
    0 -sind(r) cosd(r)];
Ry = [cosd(p) 0 -sind(p);
    0 1 0;
    sind(p) 0 cosd(p)];
Rz = [cosd(y) sind(y) 0;
    -sind(y) cosd(y) 0;
    0 0 1];

angle1 = (Rx*Ry*Rz)'*acc;

== matlab function SW_Avionic/ALTITUDE /MATLAB Function2 ==
  data: p input; rho output; t input
function rho = fcn(p,t)

M = 0.0289644; %kg/mol\
R = 8.31432; %Nm/molK

rho = (M*p)/(R*t);

== matlab function SW_Avionic/ALTITUDE /MATLAB Function3 ==
  data: rho input; h_AGL output; p input
function h_AGL = fcn(rho,p)
P0 = 101325; %N/m^2
g = 9.80665; %m/s^2
hg = 14; %m 
Pre = p-P0;
h = (Pre)/-(rho*g);
h_AGL = h-hg

== stateflow chart SW_Avionic/Deploy Parachute  ==
  state Prepare
  state Deploy
    entry:
    y =1;
  (default) -> Prepare
  Prepare -> Deploy : [V <0.5 & P < 10^5]
  data: y output; V input; P input

== matlab function SW_Avionic/ALTITUDE /MATLAB Function ==
  data: p input; rho output; t input
function rho = fcn(p,t)

M = 0.0289644; %kg/mol\
R = 8.31432; %Nm/molK

rho = (M*p)/(R*t);

== stateflow chart SW_Avionic/Touch Down  ==
  state Prepare
  state TouchDown
    Y = 1;
  (default) -> Prepare
  Prepare -> TouchDown : [V<0.5 & P>=1]
  data: P input; V input; Y output

== matlab function SW_Avionic/ALTITUDE /MATLAB Function1 ==
  data: rho input; h_AGL output; p input; Pre output
function [h_AGL, Pre]= fcn(rho,p)
P0 = 101325; %N/m^2
g = 9.80665; %m/s^2
hg = 0; %m 
Pre = p-P0;
h = (Pre)/-(rho*g);
h_AGL = h-hg

== matlab function SW_Avionic/GPS/MATLAB Function1 ==
  data: raw_val input; y output
function y = fcn(raw_val)
decimal_val = raw_val/100;
degrees = fix(decimal_val)
mm_mmmm =(decimal_val-fix(decimal_val))/0.6
y = degrees +mm_mmmm;

== matlab function SW_Avionic/GPS/MATLAB Function2 ==
  data: raw_val input; y output
function y = fcn(raw_val)
decimal_val = raw_val/100;
degrees = fix(decimal_val)
mm_mmmm =(decimal_val-fix(decimal_val))/0.6
y = degrees +mm_mmmm;

== matlab function SW_Avionic/Kalman Filter /MATLAB Function ==
  data: Qd output; R output; Ts output
function [Qd,R,Ts] = fcn()


Ts  = 0.01;
Qc = 1e-6*diag([1 1 1]);
Qd  =Qc*Ts;
R = 1e-1*diag([1 1]);

== matlab function SW_Avionic/Kalman Filter /MATLAB Function1 ==
  data: Ts input; x_est output; uk input; yp input; dh input; Qd input; R input
function x_est  = fcn(Ts,uk,yp,dh,Qd,R)

persistent X_est_p P
if isempty(X_est_p)
    X_est_p = [33 0 0]';
    P = eye(3);
end
A = [0 1 0;0 0 1;0 0 0];
B = [0 1 0]';
C = [1 0 0;0 1 0];
Ak = eye(3) + A*Ts ; 
Bk = B*Ts;
Ck = C;
%compute kalman Gain 
wk = (P*Ck')/(Ck*P*Ck'+R);
%Update predicted value 
y_est = Ck*X_est_p;
x = X_est_p + wk*([yp;dh] - y_est);
%compute predicttion at the next time step 
x_est = Ak*x + Bk*uk;
%Update covarinace matrices
P = P - wk*Ck*P;
P = Ak*P*Ak' + Qd;
X_est_p = x_est;
